simulink model "pathplanning_checkcopy"  (R2020b)
settings: Solver=FixedStepAuto  StartTime=0.0  StopTime=inf  FixedStep=0.01  RelTol=1e-3
values from neighbouring files (symbols this model uses):
  cc = cc+1    (= 1)    [Path_planning_run.m]    (also in checkpathplaning.m)
  f_stateg = 0    [Path_planning_run.m]    (also in checkpathplaning.m)
  f_statet = 270    [Path_planning_run.m]    (also in checkpathplaning.m = 180)
  f_statex = 60    [Path_planning_run.m]    (also in checkpathplaning.m = 20)
  f_statey = 64    [Path_planning_run.m]    (also in checkpathplaning.m = 40)
  gammad = [-21 0 21]    [Path_planning_run.m]    (also in checkpathplaning.m)
  i_stateg = 0    [Path_planning_run.m]    (also in checkpathplaning.m)
  i_statet = 180    [Path_planning_run.m]    (also in checkpathplaning.m)
  i_statex = 250    [Path_planning_run.m]    (also in checkpathplaning.m = 200)
  i_statey = 45    [Path_planning_run.m]    (also in checkpathplaning.m = 40)
  IC_theta0 = deg2rad(i_statet)+deg2rad(i_stateg)    [Path_planning_run.m]    (also in checkpathplaning.m)
  IC_theta1 = deg2rad(i_statet)    [Path_planning_run.m]    (also in checkpathplaning.m)
  IC_x0 = x_1f-L_0b*cos(IC_theta0)    [Path_planning_run.m]    (also in checkpathplaning.m)
  IC_x1 = i_statex    (= 250)    [Path_planning_run.m]    (also in checkpathplaning.m = 200)
  IC_y0 = y_1f-L_0b*sin(IC_theta0)    [Path_planning_run.m]    (also in checkpathplaning.m)
  IC_y1 = i_statey    (= 45)    [Path_planning_run.m]    (also in checkpathplaning.m = 40)
  L_0b = 0.3    [Path_planning_run.m]    (also in boundingbox_AV.m; check3_dyn.m; checkfinal_dyn.m; checkpathplaning.m)
  L_0f = 3.8    [Path_planning_run.m]    (also in boundingbox_AV.m; check3_dyn.m; checkfinal_dyn.m; checkpathplaning.m)
  L_1f = 8.475    [Path_planning_run.m]    (also in boundingbox_AV.m; check3_dyn.m; checkfinal_dyn.m; checkpathplaning.m)
  lookahead_timeforward = 1.5    [Path_planning_run.m]    (also in checkpathplaning.m = 2)
  lookahead_timereverse = 1.5    [Path_planning_run.m]    (also in checkpathplaning.m)
  lv12_0 = hypot((oh_0b),(w_1/2))    [Path_planning_run.m]    (also in boundingbox_AV.m; check3_dyn.m; checkfinal_dyn.m; checkpathplaning.m)
  lv12_1 = hypot(oh_1b,(w_1/2))    [Path_planning_run.m]    (also in boundingbox_AV.m; check3_dyn.m; checkfinal_dyn.m; checkpathplaning.m)
  lv34_0 = hypot((w_1/2),(L_0f+oh_0f))    [Path_planning_run.m]    (also in boundingbox_AV.m; check3_dyn.m; checkfinal_dyn.m; checkpathplaning.m)
  lv34_1 = hypot((w_1/2),oh_1f)    [Path_planning_run.m]    (also in boundingbox_AV.m; check3_dyn.m; checkfinal_dyn.m; checkpathplaning.m)
  obsc = 6    [DPDscenario.m]
  oc = 0    [Path_planning_run.m]    (also in checkpathplaning.m)
  oh_0b = 0.94    [Path_planning_run.m]    (also in boundingbox_AV.m; check3_dyn.m; checkfinal_dyn.m; checkpathplaning.m)
  oh_0f = 1.5    [Path_planning_run.m]    (also in boundingbox_AV.m; check3_dyn.m; checkfinal_dyn.m; checkpathplaning.m)
  oh_1b = 5    [Path_planning_run.m]    (also in boundingbox_AV.m; check3_dyn.m; checkfinal_dyn.m; checkpathplaning.m)
  oh_1f = L_1f+1    (= 9.475)    [Path_planning_run.m]    (also in boundingbox_AV.m; check3_dyn.m; checkfinal_dyn.m; checkpathplaning.m)
  steer_ratioforward = 1    [Path_planning_run.m]    (also in checkpathplaning.m)
  steer_ratioreverse = 1    [Path_planning_run.m]    (also in checkpathplaning.m)
  steer_sensforward = 7.7    [Path_planning_run.m]    (also in checkpathplaning.m = 4)
  steer_sensreverse = 7.2    [Path_planning_run.m]    (also in checkpathplaning.m)
  v_0 = 1    [movingobstacledetection.m]
  w_1 = 2.5    [Path_planning_run.m]    (also in boundingbox_AV.m = 10; check3_dyn.m; checkfinal_dyn.m; checkpathplaning.m)
  xv_lc = [x1_lc x2_lc x3_lc x4_lc]    [Path_planning_run.m]    (also in checkpathplaning.m)
  xv_lg = [x1_lg x2_lg x3_lg x4_lg]    [Path_planning_run.m]    (also in checkpathplaning.m; h_costnewslx.m = ppround_1(xv_lg))
  xv_rv = [61.4 30 30 61.4]    [Path_planning_run.m]    (also in checkpathplaning.m)
  yv_lc = [y1_lc y2_lc y3_lc y4_lc]    [Path_planning_run.m]    (also in checkpathplaning.m)
  yv_lg = [y1_lg y2_lg y3_lg y4_lg]    [Path_planning_run.m]    (also in checkpathplaning.m; h_costnewslx.m = ppround_1(yv_lg))
  yv_rv = [20 20 70 70]    [Path_planning_run.m]    (also in checkpathplaning.m)
undefined symbols (not defined in the file or in its folder): DiscIntNeverNeededParam, g, gfin, gini, obsx, obsy, tfin, timeAV, tini, x, xfin, y, yfin
libraries: vrlib x2, simulink x1
(part 1 of 2)
settings Model: Creator=KGMS  LastModifiedBy=KGMS

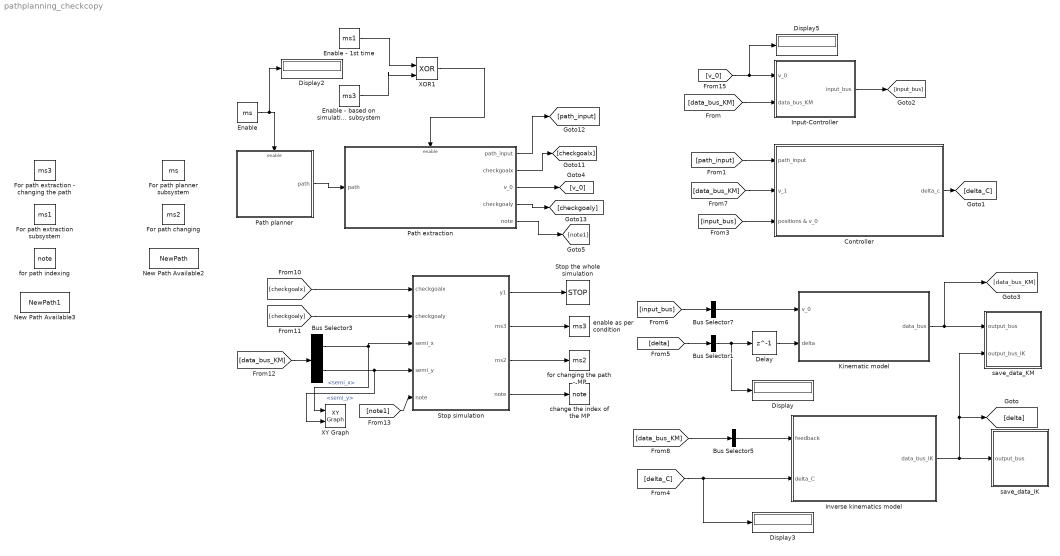
== system pathplanning_checkcopy ==
  Bus Selector1 : BusSelector  OutputSignals=angle.steering_angle  OutputAsBus=on
  Bus Selector3 : BusSelector  OutputSignals=pos.semi_x,pos.semi_y
  Bus Selector5 : BusSelector  OutputSignals=vel.velocity_semi,angle.articulation_angle  OutputAsBus=on
  Bus Selector7 : BusSelector  OutputSignals=velocity  OutputAsBus=on
  Controller : Subsystem
  Delay : Delay  DelayLength=1
  Display{,2..3,5} (4 alike) : Display
  Enable : DataStoreRead  DataStoreName=ms
  Enable - 1st time : DataStoreRead  DataStoreName=ms1
  Enable - based on simulation subsystem : DataStoreRead  DataStoreName=ms3
  For path changing : DataStoreMemory  DataStoreName=ms2  ReadBeforeWriteMsg=warning  WriteAfterWriteMsg=warning  WriteAfterReadMsg=warning  InitialValue=1  ShowAdditionalParam=off
  For path extraction - changing the path : DataStoreMemory  DataStoreName=ms3  ReadBeforeWriteMsg=warning  WriteAfterWriteMsg=warning  WriteAfterReadMsg=warning  ShowAdditionalParam=off
  For path extraction subsystem : DataStoreMemory  DataStoreName=ms1  ReadBeforeWriteMsg=warning  WriteAfterWriteMsg=warning  WriteAfterReadMsg=warning  ShowAdditionalParam=off
  For path planner subsystem : DataStoreMemory  DataStoreName=ms  ReadBeforeWriteMsg=warning  WriteAfterWriteMsg=warning  WriteAfterReadMsg=warning  InitialValue=newone  ShowAdditionalParam=off
  Input-Controller : Subsystem
  Inverse kinematics model : Subsystem
  Kinematic model : Subsystem
  New Path Available2 : DataStoreMemory  DataStoreName=NewPath  ReadBeforeWriteMsg=warning  WriteAfterWriteMsg=warning  WriteAfterReadMsg=warning  VectorParams1D=off  ShowAdditionalParam=off
  New Path Available3 : DataStoreMemory  DataStoreName=NewPath1  ReadBeforeWriteMsg=warning  WriteAfterWriteMsg=warning  WriteAfterReadMsg=warning  VectorParams1D=off  ShowAdditionalParam=off
  Path extraction : Subsystem
  Path planner : Subsystem
  Stop simulation : MATLAB Function  TreatAsAtomicUnit=on
  Stop the whole simulation : Stop
  XOR1 : Logic  Operator=XOR  IconShape=distinctive  AllPortsSameDT=off  OutDataTypeStr=boolean
  XY Graph : simulink/Sinks/XY Graph  xmin=0  xmax=286  ymin=0  ymax=80  st=-1
  change the index of the MP : DataStoreWrite  DataStoreName=note
  enable as per condition : DataStoreWrite  DataStoreName=ms3
  for changing the path - MP : DataStoreWrite  DataStoreName=ms2
  for path indexing : DataStoreMemory  DataStoreName=note  ReadBeforeWriteMsg=warning  WriteAfterWriteMsg=warning  WriteAfterReadMsg=warning  InitialValue=1  ShowAdditionalParam=off
  save_data_IK : Subsystem
  save_data_KM : Subsystem
  wires:
  Path extraction/2(checkgoalx) -> [checkgoalx]
  Delay/1 -> Kinematic model/2(delta)
  Path extraction/1(path_input) -> [path_input]
  Path extraction/3(v_0) -> [v_0]
  Kinematic model/1(data_bus) -> [data_bus_KM], save_data_KM/1(output_bus)
  [delta_C] -> Inverse kinematics model/2(delta_C), Display3/1
  Bus Selector1/1 -> Delay/1, Display/1
  [data_bus_KM] -> Bus Selector5/1
  [delta] -> Bus Selector1/1
  [v_0] -> Input-Controller/1(v_0), Display5/1
  Bus Selector7/1 -> Kinematic model/1(v_0)
  Bus Selector5/1 -> Inverse kinematics model/1(feedback)
  [path_input] -> Controller/1(path_input)
  [data_bus_KM] -> Controller/2(v_1)
  [data_bus_KM] -> Input-Controller/2(data_bus_KM)
  Path extraction/4(checkgoaly) -> [checkgoaly]
  Controller/1(delta_c) -> [delta_C]
  Path planner/1(path) -> Path extraction/1(path)
  ? -> ?
  Enable - 1st time/1 -> XOR1/1
  Enable/1 -> Path planner/Enable, Display2/1
  [input_bus] -> Controller/3(positions & v_0)
  Inverse kinematics model/1(data_bus_IK) -> save_data_IK/1(output_bus), save_data_KM/2("output_bus_IK "), [delta]
  [input_bus] -> Bus Selector7/1
  Input-Controller/1(input_bus) -> [input_bus]
  [data_bus_KM] -> Bus Selector3/1
  Bus Selector3/1 -> Stop simulation/3(semi_x), XY Graph/1  "<semi_x>"
  Bus Selector3/2 -> XY Graph/2, Stop simulation/4(semi_y)  "<semi_y>"
  Stop simulation/3(ms2) -> for changing the path - MP/1
  Stop simulation/1(y1) -> Stop the whole simulation/1
  Stop simulation/4(note) -> change the index of the MP/1
  Stop simulation/2(ms3) -> enable as per condition/1
  [checkgoaly] -> Stop simulation/2(checkgoaly)
  [checkgoalx] -> Stop simulation/1(checkgoalx)
  XOR1/1 -> Path extraction/Enable
  Enable - based on simulation subsystem/1 -> XOR1/2
  [note1] -> Stop simulation/5("note ")
  Path extraction/5(note) -> [note1]

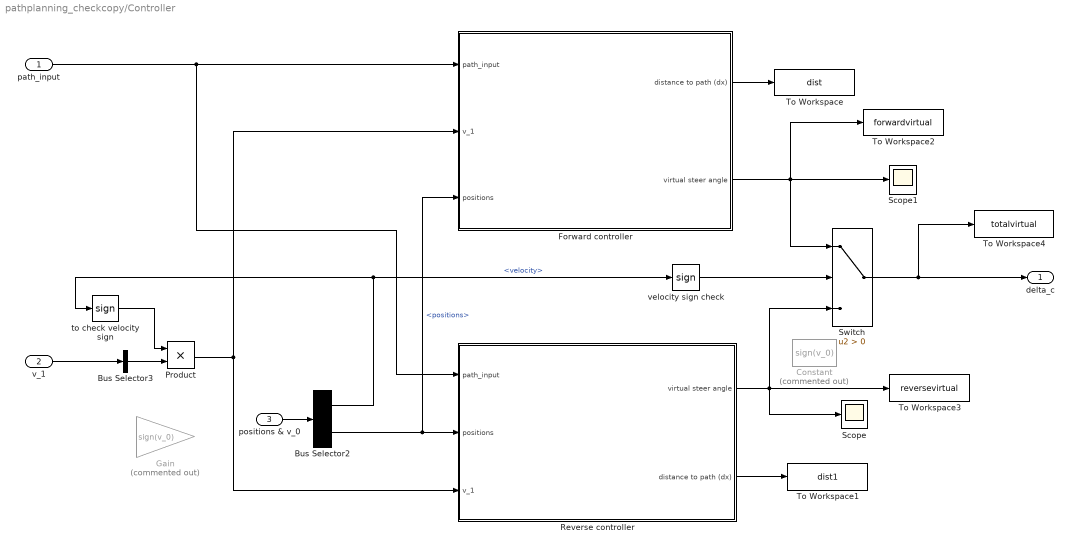
== system pathplanning_checkcopy/Controller ==
  path_input : Inport
  v_1 : Inport  Port=2
  positions & v_0 : Inport  Port=3
  Bus Selector2 : BusSelector  OutputSignals=velocity,positions
  Bus Selector3 : BusSelector  OutputSignals=vel.velocity_semi  OutputAsBus=on
  Constant : Constant  Commented=on  Value=sign(v_0)
  Forward controller : Subsystem
  Gain : Gain  Commented=on  Gain=sign(v_0)
  Product : Product
  Reverse controller : Subsystem
  Scope : Scope
  Scope1 : Scope
  Switch : Switch  Criteria=u2 > Threshold
  To Workspace : ToWorkspace  VariableName=dist  SaveFormat=Timeseries  SampleTime=-1
  To Workspace1 : ToWorkspace  VariableName=dist1  SaveFormat=Timeseries  SampleTime=-1
  To Workspace2 : ToWorkspace  VariableName=forwardvirtual  SampleTime=-1
  To Workspace3 : ToWorkspace  VariableName=reversevirtual  SampleTime=-1
  To Workspace4 : ToWorkspace  VariableName=totalvirtual  SampleTime=-1
  to check velocity sign : Signum
  velocity sign check : Signum
  delta_c : Outport
  wires:
  to check velocity sign/1 -> Product/1
  Product/1 -> Reverse controller/3(v_1), Forward controller/2(v_1)
  Forward controller/2(virtual steer angle) -> Scope1/1, To Workspace2/1, Switch/1
  path_input/1 -> Reverse controller/1(path_input), Forward controller/1(path_input)
  Bus Selector3/1 -> Product/2
  Reverse controller/1(virtual steer angle) -> To Workspace3/1, Scope/1, Switch/3
  positions & v_0/1 -> Bus Selector2/1
  Switch/1 -> delta_c/1, To Workspace4/1
  v_1/1 -> Bus Selector3/1
  velocity sign check/1 -> Switch/2
  Reverse controller/2(distance to path (dx)) -> To Workspace1/1
  Forward controller/1(distance to path (dx)) -> To Workspace/1
  Bus Selector2/2 -> Forward controller/3(positions), Reverse controller/2(positions)  "<positions>"
  Bus Selector2/1 -> to check velocity sign/1, velocity sign check/1  "<velocity>"

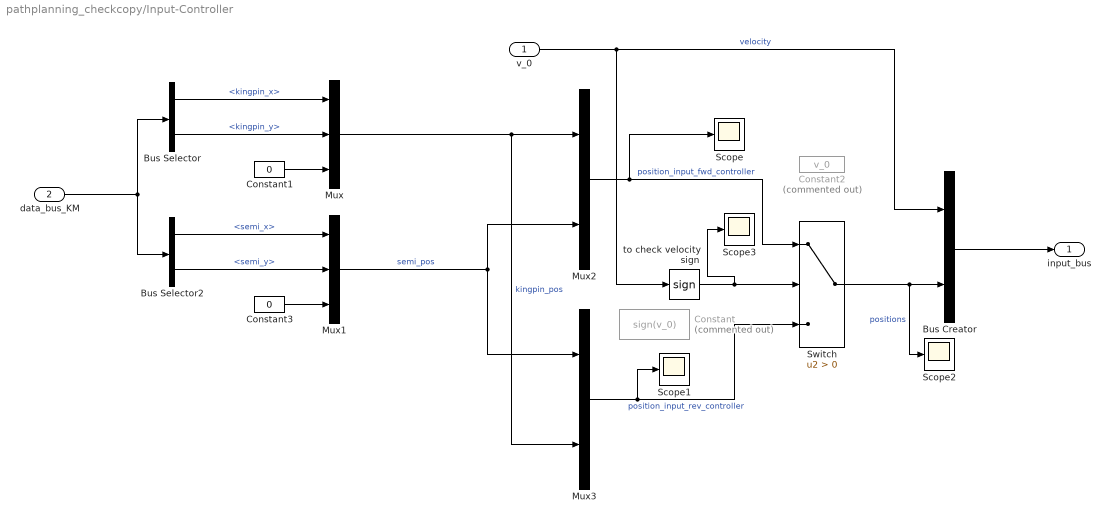
== system pathplanning_checkcopy/Input-Controller ==
  v_0 : Inport
  data_bus_KM : Inport  Port=2
  Bus Creator : BusCreator  Inputs=2
  Bus Selector : BusSelector  OutputSignals=pos.kingpin_x,pos.kingpin_y
  Bus Selector2 : BusSelector  OutputSignals=pos.semi_x,pos.semi_y
  Constant : Constant  Commented=on  Value=sign(v_0)
  Constant1 : Constant  Value=0
  Constant2 : Constant  Commented=on  Value=v_0
  Constant3 : Constant  Value=0
  Mux : Mux  Inputs=3
  Mux1 : Mux  Inputs=3
  Mux2 : Mux  Inputs=2
  Mux3 : Mux  Inputs=2
  Scope{,1..3} (4 alike) : Scope
  Switch : Switch  Criteria=u2 > Threshold
  to check velocity sign : Signum
  input_bus : Outport
  wires:
  Constant3/1 -> Mux1/3
  Bus Selector/2 -> Mux/2  "<kingpin_y>"
  Bus Selector2/1 -> Mux1/1  "<semi_x>"
  v_0/1 -> to check velocity sign/1, Bus Creator/1  "velocity"
  Bus Selector/1 -> Mux/1  "<kingpin_x>"
  Mux1/1 -> Mux3/1, Mux2/2  "semi_pos"
  Constant1/1 -> Mux/3
  Bus Selector2/2 -> Mux1/2  "<semi_y>"
  Mux/1 -> Mux3/2, Mux2/1  "kingpin_pos"
  data_bus_KM/1 -> Bus Selector2/1, Bus Selector/1
  to check velocity sign/1 -> Scope3/1, Switch/2
  Switch/1 -> Bus Creator/2, Scope2/1  "positions"
  Mux2/1 -> Switch/1, Scope/1  "position_input_fwd_controller"
  Mux3/1 -> Switch/3, Scope1/1  "position_input_rev_controller"
  Bus Creator/1 -> input_bus/1

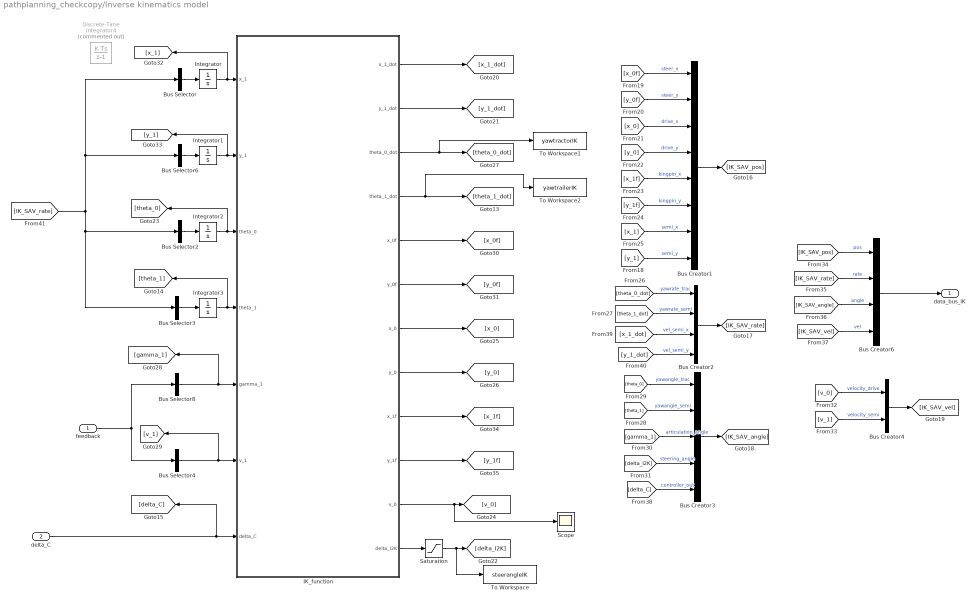
== system pathplanning_checkcopy/Inverse kinematics model ==
  feedback : Inport
  delta_C : Inport  Port=2
  Bus Creator1 : BusCreator  Inputs=8
  Bus Creator2 : BusCreator  Inputs=4
  Bus Creator3 : BusCreator  Inputs=5
  Bus Creator4 : BusCreator  Inputs=2
  Bus Creator6 : BusCreator  Inputs=4
  Bus Selector : BusSelector  OutputSignals=vel_semi_x  OutputAsBus=on
  Bus Selector2 : BusSelector  OutputSignals=yawrate_trac  OutputAsBus=on
  Bus Selector3 : BusSelector  OutputSignals=yawrate_semi  OutputAsBus=on
  Bus Selector4 : BusSelector  OutputSignals=velocity_semi  OutputAsBus=on
  Bus Selector6 : BusSelector  OutputSignals=vel_semi_y  OutputAsBus=on
  Bus Selector8 : BusSelector  OutputSignals=articulation_angle  OutputAsBus=on
  Discrete-Time Integrator4 : DiscreteIntegrator  Commented=on  InitialConditionSource=external  SampleTime=-1  ICPrevOutput=DiscIntNeverNeededParam  ICPrevScaledInput=DiscIntNeverNeededParam
  IK_function : MATLAB Function  TreatAsAtomicUnit=on
  Integrator : Integrator  InitialCondition=IC_x1
  Integrator1 : Integrator  InitialCondition=IC_y1
  Integrator2 : Integrator  InitialCondition=IC_theta0
  "Integrator3 " : Integrator  InitialCondition=IC_theta1
  Saturation : Saturate  UpperLimit=0.7  LowerLimit=-0.7
  Scope : Scope
  To Workspace : ToWorkspace  VariableName=steerangleIK  SampleTime=-1
  To Workspace1 : ToWorkspace  VariableName=yawtractorIK  SampleTime=-1
  To Workspace2 : ToWorkspace  VariableName=yawtrailerIK  SampleTime=-1
  data_bus_IK : Outport
  wires:
  IK_function/1(x_1_dot) -> [x_1_dot]
  [IK_SAV_rate] -> Bus Selector/1, Bus Selector6/1, Bus Selector3/1, Bus Selector2/1
  feedback/1 -> Bus Selector8/1, Bus Selector4/1
  IK_function/4(theta_1_dot) -> To Workspace2/1, [theta_1_dot]
  [y_1f] -> Bus Creator1/6  "kingpin_y"
  [delta_C] -> Bus Creator3/5  "controller_out"
  Bus Selector6/1 -> Integrator1/1
  IK_function/2(y_1_dot) -> [y_1_dot]
  [IK_SAV_angle] -> Bus Creator6/3  "angle"
  [y_1_dot] -> Bus Creator2/4  "vel_semi_y"
  Bus Selector4/1 -> [v_1], IK_function/6(v_1)
  Bus Creator4/1 -> [IK_SAV_vel]
  Bus Selector2/1 -> Integrator2/1
  [IK_SAV_vel] -> Bus Creator6/4  "vel"
  [y_1] -> Bus Creator1/8  "semi_y"
  [theta_1] -> Bus Creator3/2  "yawangle_semi"
  [gamma_1] -> Bus Creator3/3  "articulation_angle"
  [delta_I2K] -> Bus Creator3/4  "steering_angle"
  IK_function/5(x_0f) -> [x_0f]
  [y_0f] -> Bus Creator1/2  "steer_y"
  [IK_SAV_rate] -> Bus Creator6/2  "rate"
  IK_function/3(theta_0_dot) -> To Workspace1/1, [theta_0_dot]
  [theta_1_dot] -> Bus Creator2/2  "yawrate_semi"
  IK_function/9(x_1f) -> [x_1f]
  Bus Creator1/1 -> [IK_SAV_pos]
  [x_1_dot] -> Bus Creator2/3  "vel_semi_x"
  Bus Creator2/1 -> [IK_SAV_rate]
  [theta_0_dot] -> Bus Creator2/1  "yawrate_trac"
  Bus Creator6/1 -> data_bus_IK/1
  [x_0f] -> Bus Creator1/1  "steer_x"
  [theta_0] -> Bus Creator3/1  "yawangle_trac"
  IK_function/8(y_0) -> [y_0]
  Bus Creator3/1 -> [IK_SAV_angle]
  Bus Selector/1 -> Integrator/1
  IK_function/6(y_0f) -> [y_0f]
  [y_0] -> Bus Creator1/4  "drive_y"
  delta_C/1 -> IK_function/7(delta_C), [delta_C]
  [v_0] -> Bus Creator4/1  "velocity_drive"
  [x_0] -> Bus Creator1/3  "drive_x"
  Bus Selector3/1 -> "Integrator3 "/1
  [v_1] -> Bus Creator4/2  "velocity_semi"
  [x_1f] -> Bus Creator1/5  "kingpin_x"
  [x_1] -> Bus Creator1/7  "semi_x"
  IK_function/10(y_1f) -> [y_1f]
  Bus Selector8/1 -> [gamma_1], IK_function/5(gamma_1)
  IK_function/11(v_0) -> Scope/1, [v_0]
  IK_function/7(x_0) -> [x_0]
  Saturation/1 -> To Workspace/1, [delta_I2K]
  IK_function/12(delta_I2K) -> Saturation/1
  [IK_SAV_pos] -> Bus Creator6/1  "pos"
  Integrator/1 -> [x_1], IK_function/1(x_1)
  Integrator1/1 -> [y_1], IK_function/2(y_1)
  Integrator2/1 -> [theta_0], IK_function/3(theta_0)
  "Integrator3 "/1 -> [theta_1], IK_function/4(theta_1)

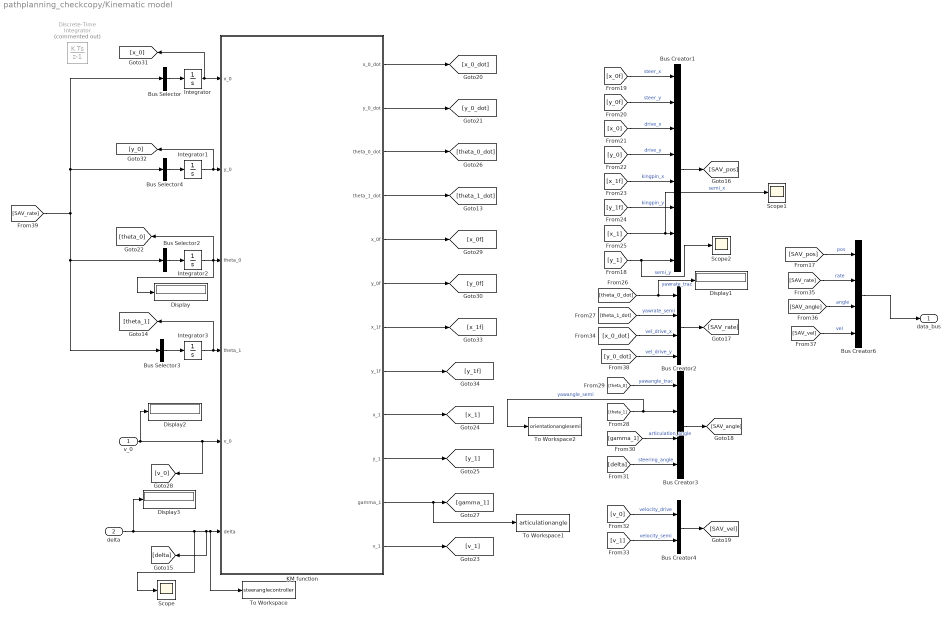
== system pathplanning_checkcopy/Kinematic model ==
  v_0 : Inport
  delta : Inport  Port=2
  Bus Creator1 : BusCreator  Inputs=8
  Bus Creator2 : BusCreator  Inputs=4
  Bus Creator3 : BusCreator  Inputs=4
  Bus Creator4 : BusCreator  Inputs=2
  Bus Creator6 : BusCreator  Inputs=4
  Bus Selector : BusSelector  OutputSignals=vel_drive_x  OutputAsBus=on
  Bus Selector2 : BusSelector  OutputSignals=yawrate_trac  OutputAsBus=on
  Bus Selector3 : BusSelector  OutputSignals=yawrate_semi  OutputAsBus=on
  Bus Selector4 : BusSelector  OutputSignals=vel_drive_y  OutputAsBus=on
  Discrete-Time Integrator : DiscreteIntegrator  Commented=on  InitialConditionSource=external  SampleTime=-1  ICPrevOutput=DiscIntNeverNeededParam  ICPrevScaledInput=DiscIntNeverNeededParam
  Display{,1..3} (4 alike) : Display
  Integrator : Integrator  InitialCondition=IC_x0
  Integrator1 : Integrator  InitialCondition=IC_y0
  Integrator2 : Integrator  InitialCondition=IC_theta0
  Integrator3 : Integrator  InitialCondition=IC_theta1
  KM function : MATLAB Function  TreatAsAtomicUnit=on
  Scope : Scope
  Scope1 : Scope
  Scope2 : Scope
  To Workspace : ToWorkspace  VariableName=steeranglecontroller  SampleTime=-1
  To Workspace1 : ToWorkspace  VariableName=articulationangle  SampleTime=-1
  To Workspace2 : ToWorkspace  VariableName=orientationanglesemi  SampleTime=-1
  data_bus : Outport
  wires:
  KM function/12(v_1) -> [v_1]
  [y_1f] -> Bus Creator1/6  "kingpin_y"
  [x_1f] -> Bus Creator1/5  "kingpin_x"
  KM function/8(y_1f) -> [y_1f]
  [x_0f] -> Bus Creator1/1  "steer_x"
  [v_1] -> Bus Creator4/2  "velocity_semi"
  [y_0f] -> Bus Creator1/2  "steer_y"
  [x_0] -> Bus Creator1/3  "drive_x"
  [x_1] -> Scope1/1, Bus Creator1/7  "semi_x"
  KM function/9(x_1) -> [x_1]
  [SAV_rate] -> Bus Selector/1, Bus Selector4/1, Bus Selector3/1, Bus Selector2/1
  KM function/2(y_0_dot) -> [y_0_dot]
  [x_0_dot] -> Bus Creator2/3  "vel_drive_x"
  Bus Creator4/1 -> [SAV_vel]
  [theta_1_dot] -> Bus Creator2/2  "yawrate_semi"
  KM function/5(x_0f) -> [x_0f]
  KM function/7(x_1f) -> [x_1f]
  KM function/10(y_1) -> [y_1]
  Bus Creator2/1 -> [SAV_rate]
  delta/1 -> Display3/1, Scope/1, [delta], To Workspace/1, KM function/6(delta)
  [y_0_dot] -> Bus Creator2/4  "vel_drive_y"
  [SAV_pos] -> Bus Creator6/1  "pos"
  KM function/3(theta_0_dot) -> [theta_0_dot]
  KM function/11(gamma_1) -> To Workspace1/1, [gamma_1]
  Bus Selector3/1 -> Integrator3/1
  v_0/1 -> Display2/1, [v_0], KM function/5(v_0)
  KM function/6(y_0f) -> [y_0f]
  [delta] -> Bus Creator3/4  "steering_angle"
  [SAV_angle] -> Bus Creator6/3  "angle"
  KM function/4(theta_1_dot) -> [theta_1_dot]
  Bus Creator3/1 -> [SAV_angle]
  Bus Selector4/1 -> Integrator1/1
  Bus Selector2/1 -> Integrator2/1
  KM function/1(x_0_dot) -> [x_0_dot]
  [SAV_vel] -> Bus Creator6/4  "vel"
  Bus Creator1/1 -> [SAV_pos]
  [theta_1] -> To Workspace2/1, Bus Creator3/2  "yawangle_semi"
  [SAV_rate] -> Bus Creator6/2  "rate"
  [v_0] -> Bus Creator4/1  "velocity_drive"
  [gamma_1] -> Bus Creator3/3  "articulation_angle"
  [y_0] -> Bus Creator1/4  "drive_y"
  [y_1] -> Scope2/1, Bus Creator1/8  "semi_y"
  [theta_0_dot] -> Display1/1, Bus Creator2/1  "yawrate_trac"
  [theta_0] -> Bus Creator3/1  "yawangle_trac"
  Bus Creator6/1 -> data_bus/1
  Bus Selector/1 -> Integrator/1
  Integrator1/1 -> [y_0], KM function/2(y_0)
  Integrator2/1 -> Display/1, [theta_0], KM function/3(theta_0)
  Integrator3/1 -> [theta_1], KM function/4(theta_1)
  Integrator/1 -> KM function/1(x_0), [x_0]

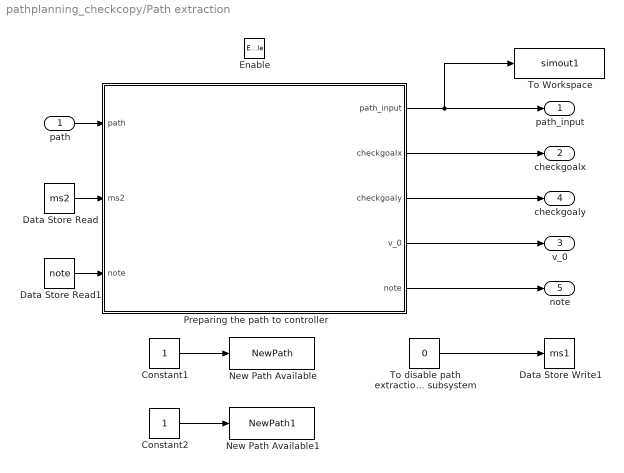
== system pathplanning_checkcopy/Path extraction ==
  path : Inport
  Enable : EnablePort
  Constant1 : Constant
  Constant2 : Constant
  Data Store Read : DataStoreRead  DataStoreName=ms2
  Data Store Read1 : DataStoreRead  DataStoreName=note
  Data Store Write1 : DataStoreWrite  DataStoreName=ms1
  New Path Available : DataStoreWrite  DataStoreName=NewPath
  New Path Available1 : DataStoreWrite  DataStoreName=NewPath1
  Preparing the path to controller : MATLAB Function  TreatAsAtomicUnit=on
  To Workspace : ToWorkspace  VariableName=simout1  SampleTime=-1
      settings: Save2DSignal=2-D array (concatenate along first dimension)
  To disable path extraction subsystem : Constant  Value=0
  path_input : Outport
  checkgoalx : Outport  Port=2
  v_0 : Outport  Port=3
  checkgoaly : Outport  Port=4
  note : Outport  Port=5
  wires:
  path/1 -> Preparing the path to controller/1(path)
  Preparing the path to controller/3(checkgoaly) -> checkgoaly/1
  To disable path extraction subsystem/1 -> Data Store Write1/1
  Preparing the path to controller/1(path_input) -> To Workspace/1, path_input/1
  Preparing the path to controller/4(v_0) -> v_0/1
  Preparing the path to controller/2(checkgoalx) -> checkgoalx/1
  Data Store Read/1 -> Preparing the path to controller/2(ms2)
  Data Store Read1/1 -> Preparing the path to controller/3("note ")
  Preparing the path to controller/5(note) -> note/1
  Constant1/1 -> New Path Available/1
  Constant2/1 -> New Path Available1/1

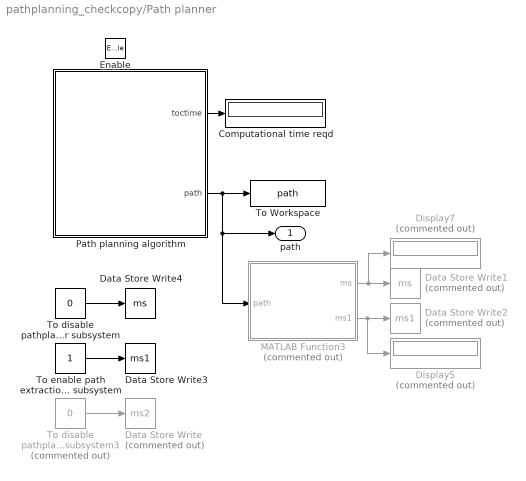
== system pathplanning_checkcopy/Path planner ==
  Enable : EnablePort
  "Computational time reqd " : Display
  Data Store Write : DataStoreWrite  Commented=on  DataStoreName=ms2
  Data Store Write1 : DataStoreWrite  Commented=on  DataStoreName=ms
  Data Store Write2 : DataStoreWrite  Commented=on  DataStoreName=ms1
  Data Store Write3 : DataStoreWrite  DataStoreName=ms1
  Data Store Write4 : DataStoreWrite  DataStoreName=ms
  Display5 : Display  Commented=on
  Display7 : Display  Commented=on
  MATLAB Function3 : MATLAB Function  Commented=on  TreatAsAtomicUnit=on
  Path planning algorithm : MATLAB Function  TreatAsAtomicUnit=on
  To Workspace : ToWorkspace  VariableName=path  SampleTime=-1
  To disable pathplanner subsystem : Constant  Value=0
  To disable pathplanner subsystem3 : Constant  Commented=on  Value=0
  To enable path extraction subsystem : Constant
  path : Outport
  wires:
  To disable pathplanner subsystem/1 -> Data Store Write4/1
  MATLAB Function3/2(ms1) -> Data Store Write2/1, Display5/1
  Path planning algorithm/2(path) -> path/1, MATLAB Function3/1(path), To Workspace/1
  MATLAB Function3/1(ms) -> Data Store Write1/1, Display7/1
  Path planning algorithm/1(toctime) -> "Computational time reqd "/1
  To enable path extraction subsystem/1 -> Data Store Write3/1
  To disable pathplanner subsystem3/1 -> Data Store Write/1

== system pathplanning_checkcopy/save_data_IK ==
  output_bus : Inport
  Bus Selector : BusSelector  OutputSignals=pos.steer_x,pos.steer_y,pos.drive_x,pos.drive_y,pos.kingpin_x,pos.kingpin_y,pos.semi_x,pos.semi_y  OutputAsBus=on
  Bus Selector1 : BusSelector  OutputSignals=rate.yawrate_trac,rate.yawrate_semi,rate.vel_semi_x,rate.vel_semi_y  OutputAsBus=on
  Bus Selector2 : BusSelector  OutputSignals=angle.yawangle_trac,angle.yawangle_semi,angle.articulation_angle,angle.steering_angle,angle.controller_out  OutputAsBus=on
  Bus Selector3 : BusSelector  OutputSignals=vel.velocity_drive,vel.velocity_semi  OutputAsBus=on
  To Workspace14 : ToWorkspace  VariableName=IK_SAV_rate  SampleTime=-1
  To Workspace15 : ToWorkspace  VariableName=IK_SAV_angle  SampleTime=-1
  To Workspace17 : ToWorkspace  VariableName=IK_SAV_vel  SampleTime=-1
  To Workspace9 : ToWorkspace  VariableName=IK_SAV_pos  SampleTime=-1
  wires:
  Bus Selector3/1 -> To Workspace17/1  "vel"
  Bus Selector/1 -> To Workspace9/1  "pos"
  Bus Selector2/1 -> To Workspace15/1  "angle"
  Bus Selector1/1 -> To Workspace14/1  "rate"
  output_bus/1 -> Bus Selector/1, Bus Selector1/1, Bus Selector3/1, Bus Selector2/1

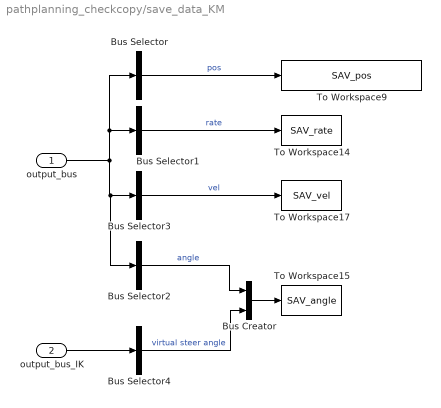
== system pathplanning_checkcopy/save_data_KM ==
  output_bus : Inport
  "output_bus_IK " : Inport  Port=2
  Bus Creator : BusCreator  Inputs=2
  Bus Selector : BusSelector  OutputSignals=pos.steer_x,pos.steer_y,pos.drive_x,pos.drive_y,pos.kingpin_x,pos.kingpin_y,pos.semi_x,pos.semi_y  OutputAsBus=on
  Bus Selector1 : BusSelector  OutputSignals=rate.yawrate_trac,rate.yawrate_semi,rate.vel_drive_x,rate.vel_drive_y  OutputAsBus=on
  Bus Selector2 : BusSelector  OutputSignals=angle.yawangle_trac,angle.yawangle_semi,angle.articulation_angle,angle.steering_angle  OutputAsBus=on
  Bus Selector3 : BusSelector  OutputSignals=vel.velocity_drive,vel.velocity_semi  OutputAsBus=on
  Bus Selector4 : BusSelector  OutputSignals=angle.controller_out  OutputAsBus=on
  To Workspace14 : ToWorkspace  VariableName=SAV_rate  SampleTime=-1
  To Workspace15 : ToWorkspace  VariableName=SAV_angle  SampleTime=-1
  To Workspace17 : ToWorkspace  VariableName=SAV_vel  SampleTime=-1
  To Workspace9 : ToWorkspace  VariableName=SAV_pos  SampleTime=-1
  wires:
  output_bus/1 -> Bus Selector2/1, Bus Selector3/1, Bus Selector1/1, Bus Selector/1
  Bus Selector1/1 -> To Workspace14/1  "rate"
  Bus Selector/1 -> To Workspace9/1  "pos"
  Bus Selector3/1 -> To Workspace17/1  "vel"
  "output_bus_IK "/1 -> Bus Selector4/1
  Bus Creator/1 -> To Workspace15/1
  Bus Selector2/1 -> Bus Creator/1  "angle"
  Bus Selector4/1 -> Bus Creator/2  "virtual steer angle"

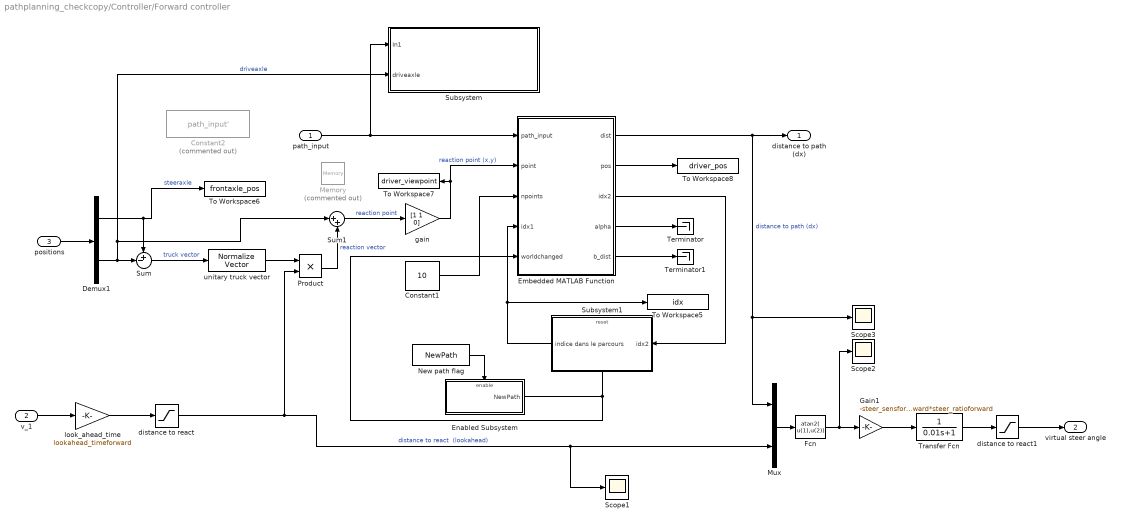
== system pathplanning_checkcopy/Controller/Forward controller ==
  path_input : Inport
  v_1 : Inport  Port=2
  positions : Inport  Port=3
  Constant1 : Constant  Value=10
  Constant2 : Constant  Commented=on  Value=path_input'
  Demux1 : Demux  Outputs=2
  Embedded MATLAB Function : MATLAB Function  TreatAsAtomicUnit=on  SystemSampleTime=[0.01 0]
  Enabled Subsystem : Subsystem  TreatAsAtomicUnit=on
  Fcn : Fcn  Expr=atan2( u(1),u(2))
  Gain1 : Gain  Gain=-steer_sensforward*steer_ratioforward
  Memory : Memory  Commented=on  InitialCondition=-1
  Mux : Mux  Inputs=2
  New path flag : DataStoreRead  DataStoreName=NewPath
  Product : Product  RndMeth=Zero
  Scope1 : Scope
  Scope2 : Scope
  Scope3 : Scope
  Subsystem : Subsystem
  Subsystem1 : Subsystem
  Sum : Sum  Inputs=+-|
  Sum1 : Sum  Inputs=|++
  Terminator : Terminator
  Terminator1 : Terminator
  To Workspace5 : ToWorkspace  VariableName=idx  SampleTime=-1
  To Workspace6 : ToWorkspace  VariableName=frontaxle_pos  SaveFormat=Structure  SampleTime=-1
  To Workspace7 : ToWorkspace  VariableName=driver_viewpoint  SaveFormat=Structure  SampleTime=-1
  To Workspace8 : ToWorkspace  VariableName=driver_pos  SampleTime=-1
  Transfer Fcn : TransferFcn  Denominator=[0.01 1]
  distance to react : Saturate  UpperLimit=100  LowerLimit=0.5
  distance to react1 : Saturate  UpperLimit=1  LowerLimit=-1
  gain : Gain  Gain=[1 1 0]
  look_ahead_time : Gain  Gain=lookahead_timeforward
  "unitary truck vector " : vrlib/Utilities/Normalize Vector  maxzero=0
  distance to path (dx) : Outport
  virtual steer angle : Outport  Port=2
  wires:
  Mux/1 -> Fcn/1
  distance to react1/1 -> virtual steer angle/1
  Product/1 -> Sum1/2  "reaction vector"
  Constant1/1 -> Embedded MATLAB Function/3(npoints)
  Demux1/1 -> To Workspace6/1, Sum/1  "steeraxle"
  Sum/1 -> "unitary truck vector "/1  "truck vector"
  Embedded MATLAB Function/1(dist) -> Mux/1, Scope3/1, distance to path (dx)/1  "distance to path (dx)"
  look_ahead_time/1 -> distance to react/1
  Embedded MATLAB Function/4(alpha) -> Terminator/1
  Fcn/1 -> Gain1/1, Scope2/1
  distance to react/1 -> Scope1/1, Mux/2, Product/2  "distance to react  (lookahead)"
  Sum1/1 -> gain/1  "reaction point"
  Embedded MATLAB Function/2(pos) -> To Workspace8/1
  "unitary truck vector "/1 -> Product/1
  gain/1 -> To Workspace7/1, Embedded MATLAB Function/2(point)  "reaction point (x,y)"
  Demux1/2 -> Subsystem/2(driveaxle), Sum1/1, Sum/2  "driveaxle"
  positions/1 -> Demux1/1
  Gain1/1 -> Transfer Fcn/1
  Embedded MATLAB Function/5(b_dist) -> Terminator1/1
  Transfer Fcn/1 -> distance to react1/1
  path_input/1 -> Embedded MATLAB Function/1(path_input), Subsystem/1(In1)
  v_1/1 -> look_ahead_time/1
  Embedded MATLAB Function/3(idx2) -> Subsystem1/1(idx2)
  New path flag/1 -> Enabled Subsystem/Enable
  Subsystem1/1(indice dans le parcours) -> To Workspace5/1, Embedded MATLAB Function/4(idx1)
  Enabled Subsystem/1(NewPath) -> Subsystem1/Reset, Embedded MATLAB Function/5(worldchanged)

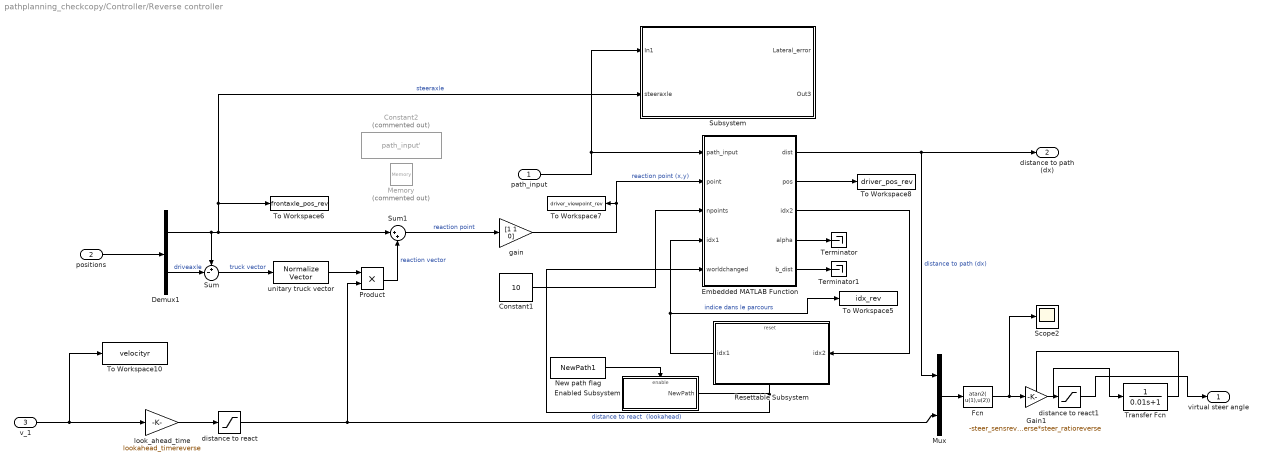
== system pathplanning_checkcopy/Controller/Reverse controller ==
  path_input : Inport
  positions : Inport  Port=2
  v_1 : Inport  Port=3
  Constant1 : Constant  Value=10
  Constant2 : Constant  Commented=on  Value=path_input'
  Demux1 : Demux  Outputs=2
  Embedded MATLAB Function : MATLAB Function  TreatAsAtomicUnit=on  SystemSampleTime=[0.01 0]
  Enabled Subsystem : Subsystem  TreatAsAtomicUnit=on
  Fcn : Fcn  Expr=atan2( u(1),u(2))
  Gain1 : Gain  Gain=-steer_sensreverse*steer_ratioreverse
  Memory : Memory  Commented=on  InitialCondition=-1
  Mux : Mux  Inputs=2
  New path flag : DataStoreRead  DataStoreName=NewPath1
  Product : Product  RndMeth=Zero
  Resettable Subsystem : Subsystem  TreatAsAtomicUnit=on
  Scope2 : Scope
  Subsystem : Subsystem
  Sum : Sum  Inputs=+-|
  Sum1 : Sum  Inputs=|++
  Terminator : Terminator
  Terminator1 : Terminator
  To Workspace10 : ToWorkspace  VariableName=velocityr  SaveFormat=Timeseries  SampleTime=-1
  To Workspace5 : ToWorkspace  VariableName=idx_rev  SampleTime=-1
  To Workspace6 : ToWorkspace  VariableName=frontaxle_pos_rev  SaveFormat=Structure  SampleTime=-1
  To Workspace7 : ToWorkspace  VariableName=driver_viewpoint_rev  SaveFormat=Structure  SampleTime=-1
  To Workspace8 : ToWorkspace  VariableName=driver_pos_rev  SampleTime=-1
  Transfer Fcn : TransferFcn  Denominator=[0.01 1]
  distance to react : Saturate  UpperLimit=100  LowerLimit=0.5
  distance to react1 : Saturate  UpperLimit=1  LowerLimit=-1
  gain : Gain  Gain=[1 1 0]
  look_ahead_time : Gain  Gain=lookahead_timereverse
  "unitary truck vector " : vrlib/Utilities/Normalize Vector  maxzero=0
  virtual steer angle : Outport
  distance to path (dx) : Outport  Port=2
  wires:
  Product/1 -> Sum1/2  "reaction vector"
  Embedded MATLAB Function/2(pos) -> To Workspace8/1
  Gain1/1 -> Transfer Fcn/1
  Embedded MATLAB Function/1(dist) -> distance to path (dx)/1, Mux/1  "distance to path (dx)"
  Demux1/1 -> Subsystem/2(steeraxle), To Workspace6/1, Sum1/1, Sum/1  "steeraxle"
  Embedded MATLAB Function/5(b_dist) -> Terminator1/1
  path_input/1 -> Embedded MATLAB Function/1(path_input), Subsystem/1(In1)
  Embedded MATLAB Function/4(alpha) -> Terminator/1
  gain/1 -> Embedded MATLAB Function/2(point), To Workspace7/1  "reaction point (x,y)"
  Transfer Fcn/1 -> distance to react1/1
  Fcn/1 -> Gain1/1, Scope2/1
  distance to react/1 -> Product/2, Mux/2  "distance to react  (lookahead)"
  Mux/1 -> Fcn/1
  Sum/1 -> "unitary truck vector "/1  "truck vector"
  "unitary truck vector "/1 -> Product/1
  Constant1/1 -> Embedded MATLAB Function/3(npoints)
  distance to react1/1 -> virtual steer angle/1
  Sum1/1 -> gain/1  "reaction point"
  v_1/1 -> look_ahead_time/1, To Workspace10/1
  Demux1/2 -> Sum/2  "driveaxle"
  look_ahead_time/1 -> distance to react/1
  positions/1 -> Demux1/1
  New path flag/1 -> Enabled Subsystem/Enable
  Enabled Subsystem/1(NewPath) -> Embedded MATLAB Function/5(worldchanged), Resettable Subsystem/Reset
  Resettable Subsystem/1(idx1) -> To Workspace5/1, Embedded MATLAB Function/4(idx1)  "indice dans le parcours"
  Embedded MATLAB Function/3(idx2) -> Resettable Subsystem/1(idx2)

== system pathplanning_checkcopy/Controller/Forward controller/Enabled Subsystem ==
  Enable : EnablePort  ZeroCross=off
  Constant : Constant
  Constant1 : Constant  Value=0
  New path flag : DataStoreWrite  DataStoreName=NewPath
  NewPath : Outport  OutputWhenDisabled=reset  InitialOutput=0  VectorParamsAs1DForOutWhenUnconnected=off
  wires:
  Constant/1 -> NewPath/1
  Constant1/1 -> New path flag/1

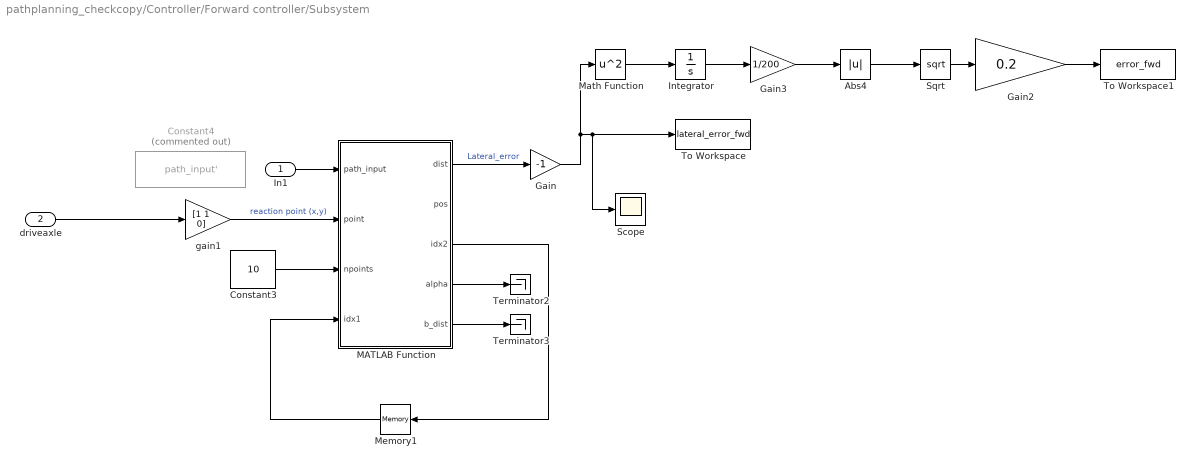
== system pathplanning_checkcopy/Controller/Forward controller/Subsystem ==
  In1 : Inport
  driveaxle : Inport  Port=2
  Abs4 : Abs
  Constant3 : Constant  Value=10
  Constant4 : Constant  Commented=on  Value=path_input'
  Gain : Gain  Gain=-1
  Gain2 : Gain  Gain=0.2
  Gain3 : Gain  Gain=1/200
  Integrator : Integrator
  MATLAB Function : MATLAB Function  TreatAsAtomicUnit=on
  Math Function : Math  Operator=square  SignedPower=on  SaturateOnIntegerOverflow=on
  Memory1 : Memory  InitialCondition=-1
  Scope : Scope
  Sqrt : Sqrt  SaturateOnIntegerOverflow=on
  Terminator2 : Terminator
  Terminator3 : Terminator
  To Workspace : ToWorkspace  VariableName=lateral_error_fwd  SampleTime=-1
  To Workspace1 : ToWorkspace  VariableName=error_fwd  SampleTime=-1
  gain1 : Gain  Gain=[1 1 0]
  wires:
  Gain/1 -> Scope/1, To Workspace/1, Math Function/1
  Abs4/1 -> Sqrt/1
  gain1/1 -> MATLAB Function/2(point)  "reaction point (x,y)"
  Gain2/1 -> To Workspace1/1
  Sqrt/1 -> Gain2/1
  Integrator/1 -> Gain3/1
  Memory1/1 -> MATLAB Function/4(idx1)
  Math Function/1 -> Integrator/1
  Gain3/1 -> Abs4/1
  MATLAB Function/1(dist) -> Gain/1  "Lateral_error"
  MATLAB Function/3(idx2) -> Memory1/1
  MATLAB Function/4(alpha) -> Terminator2/1
  MATLAB Function/5(b_dist) -> Terminator3/1
  Constant3/1 -> MATLAB Function/3(npoints)
  driveaxle/1 -> gain1/1
  In1/1 -> MATLAB Function/1(path_input)

== system pathplanning_checkcopy/Controller/Forward controller/Subsystem1 ==
  idx2 : Inport
  Reset : ResetPort  DisableCoverage=on
  Memory : Memory  InitialCondition=-1
  indice dans le parcours : Outport
  wires:
  Memory/1 -> indice dans le parcours/1  "indice dans le parcours"
  idx2/1 -> Memory/1

== system pathplanning_checkcopy/Controller/Reverse controller/Enabled Subsystem ==
  Enable : EnablePort  ZeroCross=off
  Constant : Constant
  Constant1 : Constant  Value=0
  New path flag : DataStoreWrite  DataStoreName=NewPath1
  NewPath : Outport  OutputWhenDisabled=reset  InitialOutput=0  VectorParamsAs1DForOutWhenUnconnected=off
  wires:
  Constant/1 -> NewPath/1
  Constant1/1 -> New path flag/1

== system pathplanning_checkcopy/Controller/Reverse controller/Resettable Subsystem ==
  idx2 : Inport
  Reset : ResetPort  DisableCoverage=on
  Memory : Memory  InitialCondition=-1
  idx1 : Outport
  wires:
  idx2/1 -> Memory/1
  Memory/1 -> idx1/1  "indice dans le parcours"

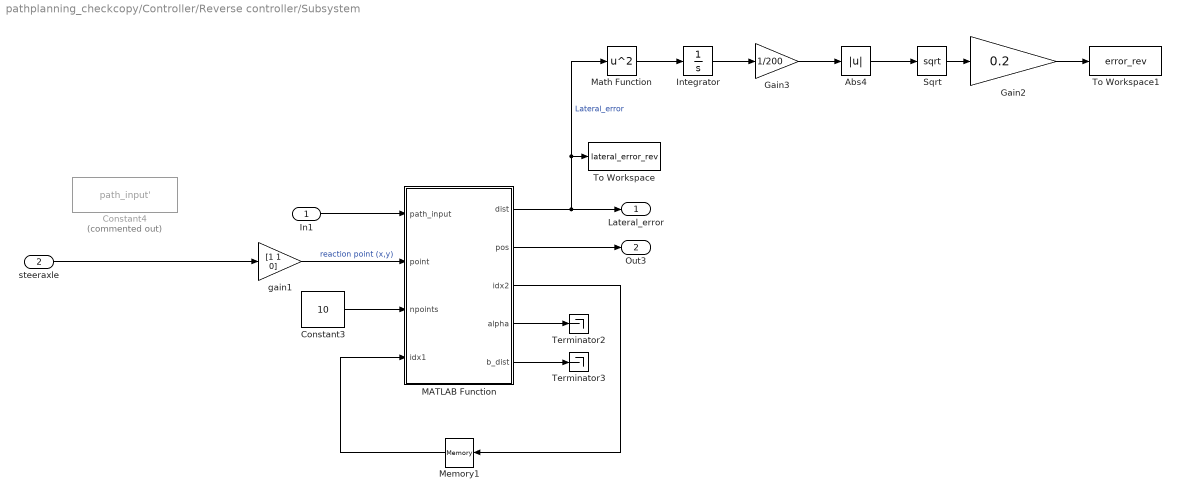
== system pathplanning_checkcopy/Controller/Reverse controller/Subsystem ==
  In1 : Inport
  steeraxle : Inport  Port=2
  Abs4 : Abs
  Constant3 : Constant  Value=10
  Constant4 : Constant  Commented=on  Value=path_input'
  Gain2 : Gain  Gain=0.2
  Gain3 : Gain  Gain=1/200
  Integrator : Integrator
  MATLAB Function : MATLAB Function  TreatAsAtomicUnit=on
  Math Function : Math  Operator=square  SignedPower=on  SaturateOnIntegerOverflow=on
  Memory1 : Memory  InitialCondition=-1
  Sqrt : Sqrt  SaturateOnIntegerOverflow=on
  Terminator2 : Terminator
  Terminator3 : Terminator
  To Workspace : ToWorkspace  VariableName=lateral_error_rev  SampleTime=-1
  To Workspace1 : ToWorkspace  VariableName=error_rev  SampleTime=-1
  gain1 : Gain  Gain=[1 1 0]
  Lateral_error : Outport
  Out3 : Outport  Port=2
  wires:
  MATLAB Function/1(dist) -> Lateral_error/1, To Workspace/1, Math Function/1  "Lateral_error"
  gain1/1 -> MATLAB Function/2(point)  "reaction point (x,y)"
  Math Function/1 -> Integrator/1
  Constant3/1 -> MATLAB Function/3(npoints)
  Sqrt/1 -> Gain2/1
  MATLAB Function/3(idx2) -> Memory1/1
  Integrator/1 -> Gain3/1
  Gain3/1 -> Abs4/1
  Memory1/1 -> MATLAB Function/4(idx1)
  In1/1 -> MATLAB Function/1(path_input)
  Abs4/1 -> Sqrt/1
  Gain2/1 -> To Workspace1/1
  MATLAB Function/5(b_dist) -> Terminator3/1
  MATLAB Function/4(alpha) -> Terminator2/1
  MATLAB Function/2(pos) -> Out3/1
  steeraxle/1 -> gain1/1

== matlab function pathplanning_checkcopy/Path extraction/Preparing the path to controller ==
  data: path_input output; path input; checkgoalx output; checkgoaly output; v_0 output; ms2 input; note input; note output
function [path_input,checkgoalx,checkgoaly,v_0,note] = fcn(path,ms2,note)
extx = nan(4000,1);
exty = nan(4000,1);
path_input = nan(4000,3);

% %__________________________________________________________________________
% % removing NaN from the path extracted
% path1 = rmmissing(path);
% path2 = path1(:,3);
% %__________________________________________________________________________
% 
% % finding the direction of vehicle
% NoMP = 21; % Resolution in motion primitives
% checkindex = length(path2)/NoMP;
% checkindex1 = 1:1:checkindex;
% c1 = nan(1,100);
% for i=1:length(checkindex1)
%     c1(:,i) = NoMP*checkindex1(i);
% end
% d1 = rmmissing(c1);
% pathdir1 = path2(d1)
% %__________________________________________________________________________
% 
% path3 = path1(:,1); % x - values
% path4 = path1(:,2); % y - values
% %new__________________-delteif dindt work__________________________________
% if ms2==1
% % Simulation - Forward path
% checkdir = pathdir1==1;
% indexdirforw = find(checkdir);
% %__________________________________________________________________________
% v_0 = 1; %velocity
% forpathx = path3((indexdirforw(1):indexdirforw(end)*21));
% forpathy = path4((indexdirforw(1):indexdirforw(end)*21));
% else
%     checkdir = pathdir1==0;
%     indexdirforw = find(checkdir);
%     v_0 = -1; %velocity
% forpathx = path3((indexdirforw(1):indexdirforw(end)*21));
% forpathy = path4((indexdirforw(1):indexdirforw(end)*21));
% end
% removing NaN from the path extracted
path1 = rmmissing(path); % remove nan's from path
MPresolution = 21;
path2 = path1(:,3); % direction
path3 = path1(:,1); % x - values
path4 = path1(:,2); % y - values
indexcheck = length(path3)/MPresolution; % total number of MP's
% index = 1:1:indexcheck; 
startdis = linspace(1,length(path3)-(MPresolution-1),indexcheck);
% startdis = round(startdis);
enddisc = linspace(21,length(path3),indexcheck);
anote = startdis(note);
enote = enddisc(note);
% enddisc = round(enddisc);
assa = ms2;
if ms2==1
%     note = index(1);
    forpathx = path3(anote:enote);
    forpathy = path4(startdis(note):enddisc(note));
    forpathv = path2(startdis(note));
else
%     note = note+1
    forpathx = path3(startdis(note):enddisc(note));
    forpathy = path4(startdis(note):enddisc(note));
    forpathv = path2(startdis(note));
%     startdis(1,:) = [];
%     enddisc(1,:) = [];
end
if forpathv==1
    v_0 = 1;% velocity
else
    v_0 = -1;
end


% 
% if ms2==1
%    checkdir = path2==1; % forward path
%    index = find(checkdir); 
%    forpathx = path3(index);
%    forpathy = path4(index);
%    v_0 = 1; % velocity
% else
%    checkdir = path2==0; % reverse path
%    index = find(checkdir); 
%    forpathx = path3(index);
%    forpathy = path4(index);
%    v_0 = -1; % velocity
% end
x_c1=pchip(linspace(1,length(forpathx),length(forpathx)),forpathx,linspace(1,length(forpathx),length(forpathx)*10)); % interpolate the x- path
y_c1=pchip(linspace(1,length(forpathy),length(forpathy)),forpathy,linspace(1,length(forpathy),length(forpathy)*10)); % interpolate the y- path
checkgoalx = x_c1(end);
checkgoaly = y_c1(end);
% x_c11 = x_c1';
% y_c11 = y_c1';
j = 10;
d_tot = 0;

while(d_tot<1.8)
    j=j+1;
    extx=interp1(linspace(1,length(x_c1),length(x_c1)),x_c1,linspace(1,length(x_c1)+(j),length(x_c1)+(j)),'linear','extrap');
    exty=interp1(linspace(1,length(y_c1),length(y_c1)),y_c1,linspace(1,length(y_c1)+(j),length(y_c1)+(j)),'linear','extrap');
%     extx=extx';
%     exty=exty';
    d = hypot(diff(extx(length(x_c1):length(extx))),diff(exty(length(y_c1):length(exty))));
    d_tot = sum (d);
end
j=length((~isnan(extx)));

% path_input(:,1) = extx;
% path_input(:,2) = exty;
% path_input(:,3) = zeros(length(path_input(:,1)),1);
path_input((1:j),1)= extx(1,(1:j));
  path_input((1:j),2) = exty(1,(1:j));% When directon changes simulate 
         path_input(:,3) = zeros(1,length(path_input(:,1)));
         note = note; % for next iteration

== matlab function pathplanning_checkcopy/Stop simulation ==
  data: checkgoalx input; y1 output; checkgoaly input; semi_x input; semi_y input; ms3 output; ms2 output; xv_lc parameter; yv_lc parameter; note output; note input
function [y1,ms3,ms2,note] = fcn(checkgoalx,checkgoaly,semi_x,semi_y,xv_lc, yv_lc,note)
ms3 =0;     % Disable Path extraction subsystem
ms2 = 1;    % Currently, keeping first index constant
% note = 1;
coder.extrinsic('InPolygon');
% areacond = false(1,1);
in = InPolygon(checkgoalx,checkgoaly,xv_lc,yv_lc); % check whether cur is in the zone
% areacond = any(in);
% if ~in && abs(checkgoalx-semi_x)<0.1 && abs(checkgoaly-semi_y)<0.1
Acheck = abs(checkgoalx-semi_x);
Bcheck = abs(checkgoaly-semi_y);
% sads = semi_x;
% asdas = semi_y;
% asdsa = checkgoalx;
% asddasdas = checkgoaly;
if ~in && Acheck<0.1 && Bcheck<0.1
    ms3 = 1 % activate path extraction subsystem for changing the path
    ms2 = 0; % activate change in path - path extraction subsystem
    y1 = 0;  % disable to stop simulation 
    note = note+1 % to update the next index to chose
%     path_input = 0;    
elseif in && Acheck<0.1 && Bcheck<0.1
    y1 = 74; % to stop the simulation
else
    ms3 = 0; % de-activate path extraction subsystem
    y1 = 0;  % disable to stop simulation
end


% while Acheck<0.1 && Bcheck<0.1
%     if ~in
%          ms1 = 1; % activate path extraction subsystem
%     ms2 = 0; % activate change in path - path extraction subsystem
%     y1 = 0;  % disable to stop simulation 
%     simfin = 0; % disable current subsystem
%     note = note+1;
%     break;
%     else
%          y1 = 74; % to stop the simulation
%     end
% end
% note = note+1;

== matlab function pathplanning_checkcopy/Controller/Forward controller/Embedded MATLAB Function ==
  settings: updateMethod=DISCRETE
  data: path_input input; point input; dist output; npoints input; pos output; idx2 output; idx1 input; alpha output; b_dist output; worldchanged input
function [dist,pos,idx2,alpha,b_dist] = dist2path(path_input,point,npoints,idx1,worldchanged)

persistent a b c idx mdist dist_sgn
path = rmmissing(path_input);
path = path';
asas = size(path);
a=[0 0 0]';
b=[0 0 0]';
c=[0 0 0]';
pos=[0 0 0]';
b_dist=[0 0 0]';
mdist=[0];
idx=0;
if worldchanged==0
idx=idx1;
end
% idx=idx1;
alpha=[0];

%Determination of idx_min and idx_max : plage de [idx-npoints,idx+npoints]
%npoints=10
if idx<0
    idx_min=1;
    idx_max=length(path);
else
    idx_min=max(1,idx-npoints);
    idx_max=min(length(path),idx+npoints);
end
% sds = idx_min
% asd = idx_max
% idx_min_dist=0;
min_dist=1e8;
ass = point;
%Determination of the shortest path to the closest reference point
for i=idx_min:idx_max
    mdist=norm(path(:,i) - point);  % Distance viewpoint to reference path for all reference points
    if mdist<min_dist               % If distance is smaller than previous distance
        idx=i;                      % Shortest path is reference point i            
        min_dist=mdist;         	% Shortest distance is updated 
        pos=path(:,i);          	% Reference point on reference path is updated.
    end
end

%Indice   Keeping reference point inside the reference path
idx=max(idx,2);
idx=min(idx,length(path)-1);


for i=idx-1:idx      
    a=path(:,i+1)-path(:,i);    %[dx dy dz] of distance between minimal ref point and previous point
    b=point-path(:,i);          % distance between reaction point and reference point
    
    b_dist=b;
    alpha=dot(a,b)/dot(a,a);    %product vectors a,b /  product vectors a,a -> rapport distance a et projection de b sur a
    dist=norm(b-alpha*a);       %distance avec la trajectoire droite entre les deux points
    
    if alpha > 0 && alpha < 1 && dist < min_dist %Le vehicule est avant le point vise  
        min_dist=dist;  %Distance mini
        pos=path(:,i)+alpha*a;  %point reellement vise
        idx=i;              
        c=cross(a,b);       %produit vectoriel  
        dist_sgn=sign(c(3));        %signe du produit vectoriel au niveau de Z
    end
end

a= path(:,idx+1) - path(:,idx);
b= point - pos;
c= cross(a,b);
dist_sgn=sign(c(3));

dist= min_dist*dist_sgn;
idx2=idx;

== matlab function pathplanning_checkcopy/Controller/Forward controller/Subsystem/MATLAB Function ==
  settings: updateMethod=DISCRETE
  data: path_input input; dist output; point input; npoints input; idx1 input; pos output; idx2 output; alpha output; b_dist output
function [dist,pos,idx2,alpha,b_dist] = dist2path(path_input,point,npoints,idx1)
%#eml
path = rmmissing(path_input);
path = path';
persistent a b c idx mdist dist_sgn

a=[0 0 0]';
b=[0 0 0]';
c=[0 0 0]';
pos=[0 0 0]';
b_dist=[0 0 0]';
mdist=[0];
idx=0;

idx=idx1;
alpha=[0];

%Determination of idx_min and idx_max : plage de [idx-npoints,idx+npoints]
%npoints=10
if idx<0
    idx_min=1;
    idx_max=length(path);
else
    idx_min=max(1,idx-npoints);
    idx_max=min(length(path),idx+npoints);
end

% idx_min_dist=0;
min_dist=1e8;

%Determination of the shortest path to the closest reference point
for i=idx_min:idx_max
    mdist=norm(path(:,i) - point);  % Distance viewpoint to reference path for all reference points
    if mdist<min_dist               % If distance is smaller than previous distance
        idx=i;                      % Shortest path is reference point i            
        min_dist=mdist;         	% Shortest distance is updated 
        pos=path(:,i);          	% Reference point on reference path is updated.
    end
end

%Indice   Keeping reference point inside the reference path
idx=max(idx,2);
idx=min(idx,length(path)-1);


for i=idx-1:idx      
    a=path(:,i+1)-path(:,i);    %[dx dy dz] of distance between minimal ref point and previous point
    b=point-path(:,i);          % distance between reaction point and reference point
    
    b_dist=b;
    alpha=dot(a,b)/dot(a,a);    %product vectors a,b /  product vectors a,a -> rapport distance a et projection de b sur a
    dist=norm(b-alpha*a);       %distance avec la trajectoire droite entre les deux points
    
    if alpha > 0 && alpha < 1 && dist < min_dist %Le vehicule est avant le point vise  
        min_dist=dist;  %Distance mini
        pos=path(:,i)+alpha*a;  %point reellement vise
        idx=i;              
        c=cross(a,b);       %produit vectoriel  
        dist_sgn=sign(c(3));        %signe du produit vectoriel au niveau de Z
    end
end

a= path(:,idx+1) - path(:,idx);
b= point - pos;
c= cross(a,b);
dist_sgn=sign(c(3));

dist= min_dist*dist_sgn;
idx2=idx;

== matlab function pathplanning_checkcopy/Inverse kinematics model/IK_function ==
  data: x_1 input; y_1 input; theta_0 input; theta_1 input; x_1_dot output; L_0b parameter; L_1f parameter; gamma_1 input; y_1_dot output; theta_0_dot output; theta_1_dot output; v_1 input; x_0f output; y_0f output; x_0 output; y_0 output; x_1f output; y_1f output; v_0 output; delta_C input; L_0f parameter; delta_I2K output
% The vehicle is described in global coordinates for which ISO system is used.
% Yaw rates can be derived from applying non-holonomic consraint (no lateral
% slip) on each axle.

function [x_1_dot,y_1_dot,theta_0_dot,theta_1_dot,x_0f,y_0f,x_0,y_0,x_1f,y_1f,...
         v_0,delta_I2K] = vehicle(x_1,y_1,theta_0,theta_1,L_0b,L_1f,gamma_1,v_1,delta_C,L_0f)
     
%_______________________ position _________________________________________
%king-pin

        x_1f = x_1+L_1f*cos(theta_1);
        y_1f = y_1+L_1f*sin(theta_1);

 
% drive axle

        x_0 = x_1f-L_0b*cos(theta_0);
        y_0 = y_1f-L_0b*sin(theta_0);

% steer axle

        x_0f = x_0+L_0f*cos(theta_0);
        y_0f = y_0+L_0f*sin(theta_0);
                       
% yaw rate        
                                      
        theta_1_dot = abs(v_1)*tan(delta_C)/L_1f;                           % semitrailer
        theta_0_dot = sign(v_1)*sign(L_0b)*(-(v_1/L_0b)*sin(gamma_1)+...
                    (L_1f/L_0b)*(theta_1_dot)*cos(gamma_1));                % tractor 
                      
% semitrailer longitudinal velocity in its own local body coordinate system

        v_0 = v_1*cos(gamma_1) + L_1f*(theta_1_dot)*sin(gamma_1); 
        
        delta_I2K = atan(L_0f*theta_0_dot/v_0);
                    
        
%_________________________next iteration___________________________________
        
        x_1_dot = v_1 * cos(theta_1);                                       % tractor drive axle velocity in global x-direction
        y_1_dot = v_1 * sin(theta_1);                                       % tractor drive axle velocity in global y-direction
